simulink model "project1"  (R2023b)
settings: Solver=VariableStepAuto  StartTime=0.0  StopTime=10.0  MaxStep=0.01  RelTol=1e-3
settings Model: Creator=mfb36  LastModifiedBy=mfb36

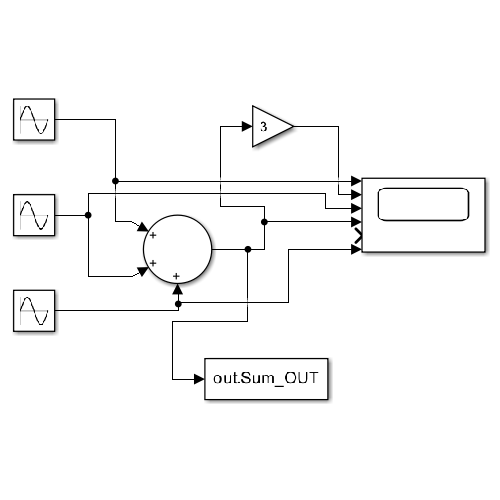
[thumbnail: Simulink's stored preview of the top-level diagram]
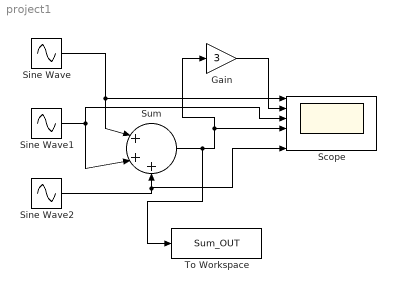
== system project1 ==
  Gain : Gain  Gain=3
  Scope : Scope  NumInputPorts=6
  Sine Wave : Sin  Amplitude=3  Frequency=5  SampleTime=0
  Sine Wave1 : Sin  Amplitude=5  SampleTime=0
  Sine Wave2 : Sin  Amplitude=10  Frequency=15  SampleTime=0
  Sum : Sum  Inputs=|+++
  To Workspace : ToWorkspace  VariableName=Sum_OUT  SaveFormat=Timeseries  SampleTime=-1
  wires:
  Sine Wave/1 -> Sum/1, Scope/1
  Sine Wave1/1 -> Sum/2, Scope/3
  Sine Wave2/1 -> Sum/3, Scope/6
  Sum/1 -> To Workspace/1, Gain/1, Scope/4
  Gain/1 -> Scope/2
